simulink model "UAV_Dynamics_Autopilot_Communication_ver2023b"  (R2023b)
settings: Solver=ode4  StartTime=0.0  StopTime=inf  FixedStep=1/1000  RelTol=1e-3
values from neighbouring files (symbols this model uses):
  dragCoeffMov = 0.01    [InitHexacopterPlantVars.m]
  m_to_mm = 1000    [InitHexacopterPlantVars.m]
  ms_to_cms = 100    [InitHexacopterPlantVars.m]
  ref_height = 23    [InitHexacopterPlantVars.m]
  ref_lat = 36.364905    [InitHexacopterPlantVars.m]
  ref_lon = 127.344377    [InitHexacopterPlantVars.m]
  rotorDir = [1 -1 1 -1 -1 1]    [InitHexacopterPlantVars.m]
  rotorPositions = zeros(3,6)    [InitHexacopterPlantVars.m]
  rotorThrustMax = 4    [InitHexacopterPlantVars.m]
  rotorTimeConst = 0.050    (= 0.05)    [InitHexacopterPlantVars.m]
  rotorTorqueMax = 0.05    [InitHexacopterPlantVars.m]
  SampleTime = 1/100    (= 0.01)    [InitHexacopterPlantVars.m]
  Ts_sensor = 1/100    (= 0.01)    [InitHexacopterPlantVars.m]
  uT_to_gauss = 0.01    [InitHexacopterPlantVars.m]
  windVel = [0 0 0]'    [InitHexacopterPlantVars.m]
  x0 = [0 0 0 0 0 0 0 0 0 0 0 0]    [InitHexacopterPlantVars.m]
undefined symbols (not defined in the file or in its folder): contact, control, ddx, ddy, ddz, dx, dy, dz, earthRadius, fractalcoef, g, Mass, p, Payload, pitch, q, r, r2d, Receive, roll, Send, X, Y, yaw, Z
libraries: uavmavlinklib x7, aerolibfltsims x3, px4MAVLinkBridgelib x2, aerolibanimutils x2, aerolibatmos2 x1, sensorgpslib x1, robotcorelib x1, mspsensorlib x1, shared6dof x1, simulink x1
settings Model: Creator=The MathWorks, Inc.  LastModifiedBy=CNU_UASG
settings SolverCC: MaxZcPerStep=1
settings ModelReferenceCC: EnableRefExpFcnMdlSchedulingChecks=on
settings RTWCC: DLArmComputeVersion=19.05

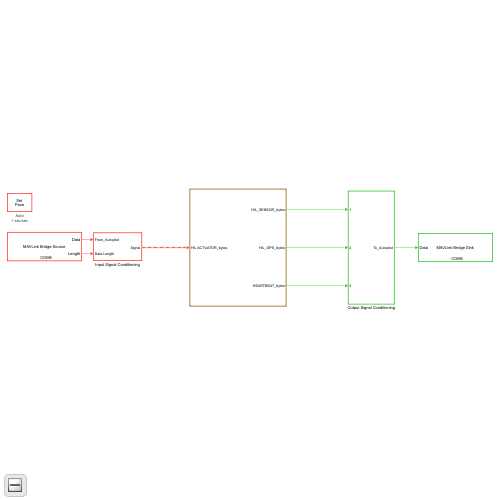
[thumbnail: Simulink's stored preview of the top-level diagram]
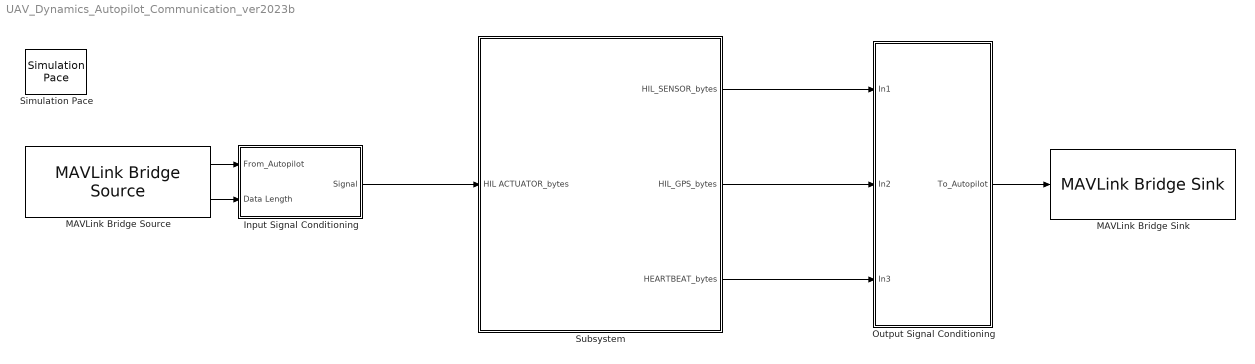
== system UAV_Dynamics_Autopilot_Communication_ver2023b ==
  Input Signal Conditioning : Subsystem
  MAVLink Bridge Sink : px4MAVLinkBridgelib/MAVLink Bridge Sink  PixhawkSerialPorttemp=Specify manually  PixhawkSerialPortManually=COM6  FieldTable={ 'UDP', '127.0.0.1', '14550' }
  MAVLink Bridge Source : px4MAVLinkBridgelib/MAVLink Bridge Source  PixhawkSerialPorttemp=Specify manually  PixhawkSerialPortManually=COM6  dataLength=MAVLink_Input_Read_Size  FieldTable={ 'UDP', '127.0.0.1', '14550' }  SampleTime=-1
  Output Signal Conditioning : Subsystem
  Simulation Pace : aerolibanimutils/Simulation Pace  SimulationPace=1  SleepMode=Auto  OutputPaceError=off  SampleTime=-1
  Subsystem : Subsystem
  wires:
  Subsystem/2(HIL_GPS_bytes) -> Output Signal Conditioning/2(In2)
  Subsystem/1(HIL_SENSOR_bytes) -> Output Signal Conditioning/1(In1)
  Subsystem/3(HEARTBEAT_bytes) -> Output Signal Conditioning/3(In3)
  Input Signal Conditioning/1(Signal) -> Subsystem/1(HIL ACTUATOR_bytes)
  MAVLink Bridge Source/1 -> Input Signal Conditioning/1(From_Autopilot)
  MAVLink Bridge Source/2 -> Input Signal Conditioning/2(Data Length)
  Output Signal Conditioning/1(To_Autopilot) -> MAVLink Bridge Sink/1

== system UAV_Dynamics_Autopilot_Communication_ver2023b/Input Signal Conditioning ==
  From_Autopilot : Inport
  Data Length : Inport  Port=2
  Constant : Constant
  Constant1 : Constant  Value=0  OutDataTypeStr=uint8  SampleTime=-1
  Data Type Conversion : DataTypeConversion  OutDataTypeStr=double  SaturateOnIntegerOverflow=off  RndMeth=Floor
  Mux1 : Mux  Inputs=2
  Reshape : Reshape
  Selector : Selector  InputPortWidth=MAVLink_Input_Read_Size  IndexOptions=Starting and ending indices (port)  Indices=[1 3]  OutputSizes=1
  Switch : Switch  Criteria=u2 > Threshold  SaturateOnIntegerOverflow=off  InputSameDT=off
  Signal : Outport
  wires:
  Reshape/1 -> Signal/1
  Mux1/1 -> Selector/2
  Data Length/1 -> Data Type Conversion/1
  Constant/1 -> Mux1/1
  Selector/1 -> Switch/1
  From_Autopilot/1 -> Selector/1
  Constant1/1 -> Switch/3
  Switch/1 -> Reshape/1
  Data Type Conversion/1 -> Switch/2, Mux1/2

== system UAV_Dynamics_Autopilot_Communication_ver2023b/Output Signal Conditioning ==
  In1 : Inport
  In2 : Inport  Port=2
  In3 : Inport  Port=3
  Mux : Mux  Inputs=3
  To_Autopilot : Outport
  wires:
  Mux/1 -> To_Autopilot/1
  In2/1 -> Mux/2
  In3/1 -> Mux/3
  In1/1 -> Mux/1

== system UAV_Dynamics_Autopilot_Communication_ver2023b/Subsystem ==
  HIL ACTUATOR_bytes : Inport  OutDataTypeStr=uint8  PortDimensions=MAVLink_Input_Read_Size  SampleTime=SampleTime  Interpolate=off
      settings: VarSizeSig=Yes
  HIL_ACTUATOR_CONTROLS : Subsystem
  HIL_GPS : Subsystem
  HIL_SENSOR : Subsystem
  Send Heartbeat : Subsystem
  Subsystem : Subsystem
  HIL_SENSOR_bytes : Outport  BusOutputAsStruct=on
  HIL_GPS_bytes : Outport  Port=2  BusOutputAsStruct=on
  HEARTBEAT_bytes : Outport  Port=3  BusOutputAsStruct=on
  wires:
  Subsystem/2(Gyro) -> HIL_SENSOR/2(Gyro)
  Subsystem/4(Pressure) -> HIL_SENSOR/4(Pressure)
  Subsystem/6(Velocity) -> HIL_GPS/2(Velocity)
  Subsystem/3(Mag) -> HIL_SENSOR/3(Mag)
  Subsystem/8(Course) -> HIL_GPS/4(Course)
  HIL_ACTUATOR_CONTROLS/1(Actuator) -> Subsystem/1(PWM Inputs)
  Subsystem/1(Acc) -> HIL_SENSOR/1(Acc)
  Subsystem/5(LLA) -> HIL_GPS/1(LLA)
  HIL_GPS/1(HIL_GPS_bytes) -> HIL_GPS_bytes/1
  HIL_SENSOR/1(HIL_SENSOR_bytes) -> HIL_SENSOR_bytes/1
  HIL ACTUATOR_bytes/1 -> HIL_ACTUATOR_CONTROLS/1(HIL ACTUATOR_bytes)
  Subsystem/7(GndSpeed) -> HIL_GPS/3(GndSpeed)
  Send Heartbeat/1(HEARTBEAT_bytes) -> HEARTBEAT_bytes/1

== system UAV_Dynamics_Autopilot_Communication_ver2023b/Subsystem/HIL_ACTUATOR_CONTROLS ==
  HIL ACTUATOR_bytes : Inport
  Bus Selector : BusSelector  OutputSignals=Payload.controls
  Data Type Conversion : DataTypeConversion  OutDataTypeStr=double  SaturateOnIntegerOverflow=off  RndMeth=Floor
  MAVLink Deserializer : uavmavlinklib/MAVLink Deserializer  dialectSource=Select from standard MAVLink dialects  dialect=common.xml  dialectCustom=common.xml  version=2  messageType=HIL_ACTUATOR_CONTROLS  inputDataLength=off  SystemIDFilter=off  systemID=1  ComponentIDFilter=off  componentID=1  queueMsg=off  queueMsgSize=50  dropNum=off
  Saturation : Saturate  UpperLimit=1  LowerLimit=0
  Selector1 : Selector  InputPortWidth=16  IndexOptions=Index vector (dialog)  Indices=[1:6]  OutputSizes=1
  Terminator : Terminator
  Actuator : Outport
  wires:
  Saturation/1 -> Actuator/1
  Selector1/1 -> Saturation/1  "Controls"
  HIL ACTUATOR_bytes/1 -> MAVLink Deserializer/1
  Bus Selector/1 -> Data Type Conversion/1  "<controls>"
  MAVLink Deserializer/2 -> Bus Selector/1
  MAVLink Deserializer/1 -> Terminator/1
  Data Type Conversion/1 -> Selector1/1

== system UAV_Dynamics_Autopilot_Communication_ver2023b/Subsystem/HIL_GPS ==
  LLA : Inport
  Velocity : Inport  Port=2
  GndSpeed : Inport  Port=3
  Course : Inport  Port=4
  HIL_GPS Subsystem : Subsystem
  MAVLink Serializer3 : uavmavlinklib/MAVLink Serializer  dialectSource=Select from standard MAVLink dialects  dialect=common.xml  dialectCustom=common.xml  version=2  messageType=HIL_GPS
  Rate Transition : RateTransition  OutPortSampleTime=Ts_sensor
  Terminator2 : Terminator
  HIL_GPS_bytes : Outport
  wires:
  Rate Transition/1 -> MAVLink Serializer3/1
  Velocity/1 -> HIL_GPS Subsystem/2(Velocity)
  MAVLink Serializer3/1 -> HIL_GPS_bytes/1
  GndSpeed/1 -> HIL_GPS Subsystem/3(GndSpeed)
  LLA/1 -> HIL_GPS Subsystem/1(LLA)
  MAVLink Serializer3/2 -> Terminator2/1
  Course/1 -> HIL_GPS Subsystem/4(Course)
  HIL_GPS Subsystem/1(Out1) -> Rate Transition/1

== system UAV_Dynamics_Autopilot_Communication_ver2023b/Subsystem/HIL_SENSOR ==
  Acc : Inport
  Gyro : Inport  Port=2
  Mag : Inport  Port=3
  Pressure : Inport  Port=4
  HIL_SENSOR Creation subsystem : Subsystem
  MAVLink Serializer1 : uavmavlinklib/MAVLink Serializer  dialectSource=Select from standard MAVLink dialects  dialect=common.xml  dialectCustom=common.xml  version=2  messageType=HIL_SENSOR
  Rate Transition : RateTransition  OutPortSampleTime=Ts_sensor
  Terminator : Terminator
  HIL_SENSOR_bytes : Outport
  wires:
  Rate Transition/1 -> MAVLink Serializer1/1
  Gyro/1 -> HIL_SENSOR Creation subsystem/2(Gyro)
  HIL_SENSOR Creation subsystem/1(HIL Sensor) -> Rate Transition/1
  Mag/1 -> HIL_SENSOR Creation subsystem/3(Mag)
  MAVLink Serializer1/1 -> HIL_SENSOR_bytes/1
  MAVLink Serializer1/2 -> Terminator/1
  Acc/1 -> HIL_SENSOR Creation subsystem/1(Acc)
  Pressure/1 -> HIL_SENSOR Creation subsystem/4(Pressure)

== system UAV_Dynamics_Autopilot_Communication_ver2023b/Subsystem/Send Heartbeat ==
  Bus Assignment : BusAssignment  AssignedSignals=Payload.autopilot,Payload.type
  Constant : Constant  SampleTime=-1
  Constant1 : Constant  Value=12  SampleTime=-1
  Data Type Conversion : DataTypeConversion  OutDataTypeStr=uint8  SaturateOnIntegerOverflow=off  RndMeth=Floor
  Data Type Conversion1 : DataTypeConversion  OutDataTypeStr=uint8  SaturateOnIntegerOverflow=off  RndMeth=Floor
  MAVLink Blank Message : uavmavlinklib/MAVLink Blank Message  dialectSource=Select from standard MAVLink dialects  dialect=common.xml  dialectCustom=common.xml  version=2  messageType=HEARTBEAT  SystemID=2  ComponentID=51  SampleTime=Ts_sensor
  MAVLink Serializer : uavmavlinklib/MAVLink Serializer  dialectSource=Select from standard MAVLink dialects  dialect=common.xml  dialectCustom=common.xml  version=2  messageType=HEARTBEAT
  Terminator4 : Terminator
  HEARTBEAT_bytes : Outport
  wires:
  MAVLink Blank Message/1 -> Bus Assignment/1
  Constant1/1 -> Data Type Conversion1/1
  MAVLink Serializer/2 -> Terminator4/1
  Data Type Conversion/1 -> Bus Assignment/2
  Data Type Conversion1/1 -> Bus Assignment/3
  MAVLink Serializer/1 -> HEARTBEAT_bytes/1
  Constant/1 -> Data Type Conversion/1
  Bus Assignment/1 -> MAVLink Serializer/1

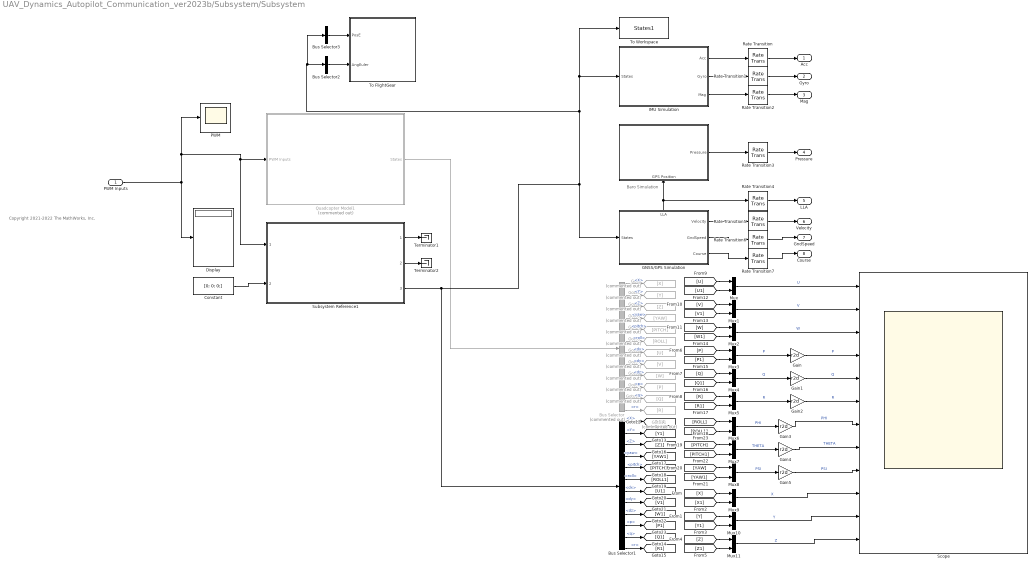
== system UAV_Dynamics_Autopilot_Communication_ver2023b/Subsystem/Subsystem ==
  note: Baro Simulation
  note: Copyright 2021-2022 The MathWorks, Inc.
  PWM Inputs : Inport
  " " : Subsystem
      settings: PortSchema="{\"entries\":[{\"content\":{\"sides\":[{\"content\":{\"connectorIds\":[]},\"type\":\"ConnectorPlacement.EquallySpacedRectSide\",\"uuid\":\"7ecc8b21-8f8f-4144-826a-6b68e30dbf7d\"},{\"content\":{\"connectorIds\":[\"Out1\"],\"side\":\"RIGHT\"},\"type\":\"ConnectorPlacement.EquallySpacedRectSide\",\"uuid\":\"81a1dd55-8330-4386-9921-36c0eb60d526\"},{\"content\":{\"connectorIds\":[],\"side\":\"TOP\"},\"type\":\"ConnectorPlacement.EquallySpacedRectSide\",\"uuid\":\"b99caff5-b40d-407d-b30e-35210c1aee1d\"},{\"content\":{\"connectorIds\":[\"In1\"],\"side\":\"BOTTOM\"},\"type\":\"ConnectorPlacement.EquallySpacedRectSide\",\"uuid\":\"18bfda3d-4fab-4e61-9ebc-e384e51de306\"}]},\"type\":\"ConnectorPlacement.EquallySpacedConnector\",\"uuid\":\"17ab4e96-b761-4c62-a0bb-ab626dac3eaa\"}],\"packageUris\":[\"http://schema.mathworks.com/mf0/Connector/R2020b\"],\"version\":\"1.0\"}"
  Bus Selector : BusSelector  Commented=on  OutputSignals=X,Y,Z,yaw,pitch,roll,dx,dy,dz,p,q,r
  Bus Selector1 : BusSelector  OutputSignals=X,Y,Z,yaw,pitch,roll,dx,dy,dz,p,q,r
  Bus Selector2 : BusSelector  OutputSignals=roll,pitch,yaw  OutputAsBus=on
  Bus Selector3 : BusSelector  OutputSignals=X,Y,Z  OutputAsBus=on
  Constant : Constant  Value=[0; 0; 0;]
  Display : Display
  GNSS/GPS Simulation : Subsystem
      settings: PortSchema="{\"entries\":[{\"content\":{\"sides\":[{\"content\":{\"connectorIds\":[\"In1\"]},\"type\":\"ConnectorPlacement.EquallySpacedRectSide\",\"uuid\":\"4934e8ff-5d4b-4e11-968d-c23bd62383a0\"},{\"content\":{\"connectorIds\":[\"Out1\",\"Out2\",\"Out3\"],\"side\":\"RIGHT\"},\"type\":\"ConnectorPlacement.EquallySpacedRectSide\",\"uuid\":\"9ec8bc0a-2d3c-4dca-835c-010ac29b6ebc\"},{\"content\":{\"connectorIds\":[\"Out4\"],\"side\":\"TOP\"},\"type\":\"ConnectorPlacement.EquallySpacedRectSide\",\"uuid\":\"04f09eb4-1bd9-450e-b951-47054bdd92ad\"}]},\"type\":\"ConnectorPlacement.EquallySpacedConnector\",\"uuid\":\"9a5920cf-a58d-4c98-839b-fbac94edbe7e\"}],\"packageUris\":[\"http://schema.mathworks.com/mf0/Connector/R2020b\"],\"version\":\"1.0\"}"
  Gain{,1..5} (6 alike) : Gain  Gain=r2d
  Goto : Goto  Commented=on  GotoTag=X
  Goto1 : Goto  Commented=on  GotoTag=Y
  Goto10 : Goto  Commented=on  GotoTag=Q
  Goto11 : Goto  Commented=on  GotoTag=R
  Goto2 : Goto  Commented=on  GotoTag=Z
  Goto3 : Goto  Commented=on  GotoTag=YAW
  Goto4 : Goto  Commented=on  GotoTag=PITCH
  Goto5 : Goto  Commented=on  GotoTag=ROLL
  Goto6 : Goto  Commented=on  GotoTag=U
  Goto7 : Goto  Commented=on  GotoTag=V
  Goto8 : Goto  Commented=on  GotoTag=W
  Goto9 : Goto  Commented=on  GotoTag=P
  IMU Simulation : Subsystem
  Mux{,1..11} (12 alike) : Mux  Inputs=2
  PWM : Scope
  Quadcopter Model1 : Subsystem  Commented=on
  Rate Transition{,1..7} (8 alike) : RateTransition  OutPortSampleTime=Ts_sensor
  Scope : Scope  NumInputPorts=12
  Subsystem Reference1 : Subsystem  ReferencedSubsystem=F550_Dynamics_sub_ver2023b
  Terminator1 : Terminator
  Terminator2 : Terminator
  To FlightGear : Subsystem
      mask Display: image('79904309.png');
  To Workspace : ToWorkspace  VariableName=States1  SaveFormat=Structure With Time  SampleTime=-1
  Acc : Outport
  Gyro : Outport  Port=2
  Mag : Outport  Port=3
  Pressure : Outport  Port=4
  LLA : Outport  Port=5
  Velocity : Outport  Port=6
  GndSpeed : Outport  Port=7
  Course : Outport  Port=8
  wires:
  Subsystem Reference1/1 -> Terminator1/1
  Bus Selector/8 -> Goto7/1  "<dy>"
  [PITCH1] -> Mux7/2
  Mux2/1 -> Scope/3  "W"
  Bus Selector1/1 -> [X1]  "<X>"
  GNSS/GPS Simulation/2(GndSpeed) -> Rate Transition6/1
  [YAW1] -> Mux8/2
  [X] -> Mux9/1
  GNSS/GPS Simulation/1(Velocity) -> Rate Transition5/1
  PWM Inputs/1 -> Display/1, PWM/1, Quadcopter Model1/1(PWM Inputs), Subsystem Reference1/1
  [PITCH] -> Mux7/1
  [YAW] -> Mux8/1
  [X1] -> Mux9/2
  Bus Selector/12 -> Goto11/1  "<r>"
  Bus Selector1/2 -> [Y1]  "<Y>"
  GNSS/GPS Simulation/3(Course) -> Rate Transition7/1
  Constant/1 -> Subsystem Reference1/2
  Bus Selector1/5 -> [PITCH1]  "<pitch>"
  Bus Selector/3 -> Goto2/1  "<Z>"
  Bus Selector/6 -> Goto5/1  "<roll>"
  Bus Selector1/4 -> [YAW1]  "<yaw>"
  Mux8/1 -> Gain5/1  "PSI"
  Bus Selector1/12 -> [R1]  "<r>"
  IMU Simulation/2(Gyro) -> Rate Transition1/1
  [P] -> Mux3/1
  [U1] -> Mux/2
  [Q1] -> Mux4/2
  [Y1] -> Mux10/2
  [Z] -> Mux11/1
  Bus Selector/11 -> Goto10/1  "<q>"
  Bus Selector/7 -> Goto6/1  "<dx>"
  Bus Selector/5 -> Goto4/1  "<pitch>"
  Bus Selector/1 -> Goto/1  "<X>"
  Bus Selector/4 -> Goto3/1  "<yaw>"
  Bus Selector1/10 -> [P1]  "<p>"
  [Z1] -> Mux11/2
  Bus Selector/10 -> Goto9/1  "<p>"
  [V1] -> Mux1/2
  Mux7/1 -> Gain4/1  "THETA"
  [R] -> Mux5/1
  " "/1(Pressure) -> Rate Transition3/1
  [W1] -> Mux2/2
  [P1] -> Mux3/2
  GNSS/GPS Simulation/4(LLA) -> " "/1(GPS Position), Rate Transition4/1
  [Q] -> Mux4/1
  Bus Selector1/8 -> [V1]  "<dy>"
  [Y] -> Mux10/1
  Bus Selector3/1 -> To FlightGear/1(PosE)
  Subsystem Reference1/2 -> Terminator2/1
  [V] -> Mux1/1
  [W] -> Mux2/1
  [ROLL] -> Mux6/1
  Mux/1 -> Scope/1  "U"
  Mux10/1 -> Scope/11  "Y"
  Bus Selector1/9 -> [W1]  "<dz>"
  [R1] -> Mux5/2
  Mux1/1 -> Scope/2  "V"
  Mux4/1 -> Gain1/1  "Q"
  Mux6/1 -> Gain3/1  "PHI"
  Mux3/1 -> Gain/1  "P"
  Mux9/1 -> Scope/10  "X"
  Bus Selector/2 -> Goto1/1  "<Y>"
  Bus Selector1/11 -> [Q1]  "<q>"
  Bus Selector1/6 -> [ROLL1]  "<roll>"
  [ROLL1] -> Mux6/2
  Mux11/1 -> Scope/12  "Z"
  IMU Simulation/1(Acc) -> Rate Transition/1
  IMU Simulation/3(Mag) -> Rate Transition2/1
  Bus Selector2/1 -> To FlightGear/2(AngEuler)
  [U] -> Mux/1
  Bus Selector1/3 -> [Z1]  "<Z>"
  Bus Selector/9 -> Goto8/1  "<dz>"
  Bus Selector1/7 -> [U1]  "<dx>"
  Quadcopter Model1/1(States) -> Bus Selector/1
  Mux5/1 -> Gain2/1  "R"
  Gain/1 -> Scope/4  "P"
  Gain1/1 -> Scope/5  "Q"
  Gain2/1 -> Scope/6  "R"
  Gain3/1 -> Scope/7  "PHI"
  Gain4/1 -> Scope/8  "THETA"
  Gain5/1 -> Scope/9  "PSI"
  Subsystem Reference1/3 -> GNSS/GPS Simulation/1(States), IMU Simulation/1(States), To Workspace/1, Bus Selector2/1, Bus Selector3/1, Bus Selector1/1
  Rate Transition/1 -> Acc/1
  Rate Transition1/1 -> Gyro/1
  Rate Transition2/1 -> Mag/1
  Rate Transition3/1 -> Pressure/1
  Rate Transition4/1 -> LLA/1
  Rate Transition5/1 -> Velocity/1
  Rate Transition7/1 -> Course/1
  Rate Transition6/1 -> GndSpeed/1

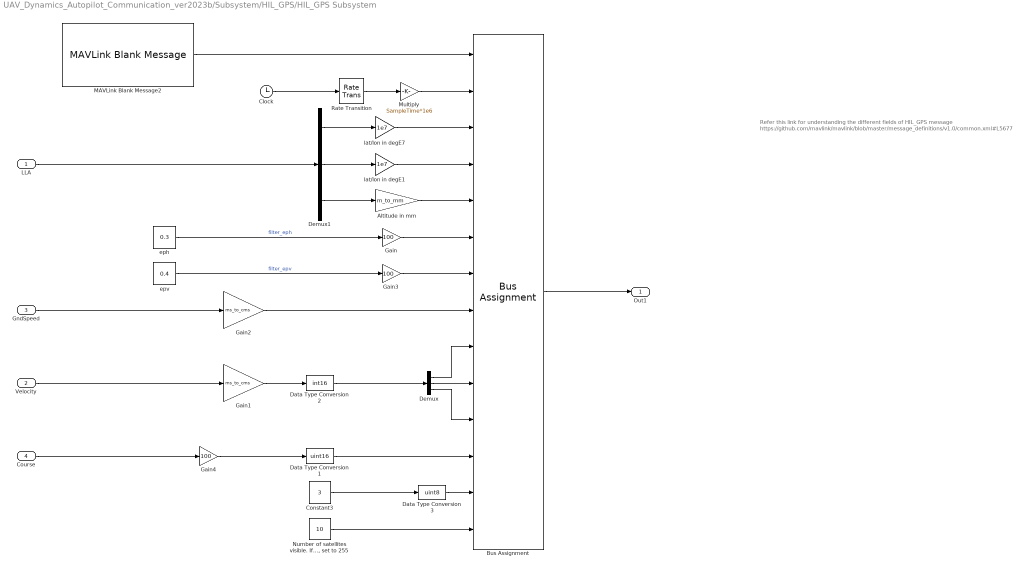
== system UAV_Dynamics_Autopilot_Communication_ver2023b/Subsystem/HIL_GPS/HIL_GPS Subsystem ==
  note: Refer this link for understanding the different fields of HIL_GPS message https://github.com/mavlink/mavlink/blob/master/message_definitions/v1.0/common.xml#L5677
  LLA : Inport
  Velocity : Inport  Port=2
  GndSpeed : Inport  Port=3
  Course : Inport  Port=4
  Altitude in mm : Gain  Gain=m_to_mm  OutDataTypeStr=Inherit: Inherit via back propagation
  Bus Assignment : BusAssignment  AssignedSignals=Payload.time_usec,Payload.lat,Payload.lon,Payload.alt,Payload.eph,Payload.epv,Payload.vel,Payload.vn,Payload.ve,Payload.vd,Payload.cog,Payload.fix_type,Payload.satellites_visible
  Clock : Clock
  Constant3 : Constant  Value=3  OutDataTypeStr=Inherit: Inherit via back propagation  SampleTime=Ts_sensor
  Data Type Conversion1 : DataTypeConversion  OutDataTypeStr=uint16  SaturateOnIntegerOverflow=off  RndMeth=Floor
  Data Type Conversion2 : DataTypeConversion  OutDataTypeStr=int16  SaturateOnIntegerOverflow=off  RndMeth=Floor
  Data Type Conversion3 : DataTypeConversion  OutDataTypeStr=uint8  SaturateOnIntegerOverflow=off  RndMeth=Floor
  Demux : Demux  Outputs=3
  Demux1 : Demux  Outputs=3
  Gain : Gain  Gain=100  OutDataTypeStr=Inherit: Inherit via back propagation
  Gain1 : Gain  Gain=ms_to_cms
  Gain2 : Gain  Gain=ms_to_cms  OutDataTypeStr=uint16
  Gain3 : Gain  Gain=100  OutDataTypeStr=Inherit: Inherit via back propagation
  Gain4 : Gain  Gain=100
  MAVLink Blank Message2 : uavmavlinklib/MAVLink Blank Message  dialectSource=Select from standard MAVLink dialects  dialect=common.xml  dialectCustom=common.xml  version=2  messageType=HIL_GPS  SystemID=2  ComponentID=51  SampleTime=Ts_sensor
  Multiply : Gain  Gain=SampleTime*1e6  OutDataTypeStr=Inherit: Inherit via back propagation
  "Number of satellites visible. If unknown, set to 255" : Constant  Value=10  OutDataTypeStr=Inherit: Inherit via back propagation  SampleTime=Ts_sensor
  Rate Transition : RateTransition  OutPortSampleTime=Ts_sensor
  eph : Constant  Value=0.3  SampleTime=Ts_sensor
  epv : Constant  Value=0.4  SampleTime=Ts_sensor
  lat/lon in degE1 : Gain  Gain=1e7  OutDataTypeStr=Inherit: Inherit via back propagation
  lat/lon in degE7 : Gain  Gain=1e7  OutDataTypeStr=Inherit: Inherit via back propagation
  Out1 : Outport
  wires:
  Multiply/1 -> Bus Assignment/2
  Rate Transition/1 -> Multiply/1
  Clock/1 -> Rate Transition/1
  Constant3/1 -> Data Type Conversion3/1
  Gain4/1 -> Data Type Conversion1/1
  Data Type Conversion3/1 -> Bus Assignment/13
  epv/1 -> Gain3/1  "filter_epv"
  eph/1 -> Gain/1  "filter_eph"
  Data Type Conversion1/1 -> Bus Assignment/12
  Course/1 -> Gain4/1
  Velocity/1 -> Gain1/1
  GndSpeed/1 -> Gain2/1
  LLA/1 -> Demux1/1
  Gain3/1 -> Bus Assignment/7
  Gain/1 -> Bus Assignment/6
  "Number of satellites visible. If unknown, set to 255"/1 -> Bus Assignment/14
  Bus Assignment/1 -> Out1/1
  Demux/2 -> Bus Assignment/10
  Data Type Conversion2/1 -> Demux/1
  Altitude in mm/1 -> Bus Assignment/5
  lat/lon in degE1/1 -> Bus Assignment/4
  Demux/1 -> Bus Assignment/9
  Demux1/2 -> lat/lon in degE1/1
  Demux1/3 -> Altitude in mm/1
  Gain1/1 -> Data Type Conversion2/1
  MAVLink Blank Message2/1 -> Bus Assignment/1
  Demux/3 -> Bus Assignment/11
  Demux1/1 -> lat/lon in degE7/1
  lat/lon in degE7/1 -> Bus Assignment/3
  Gain2/1 -> Bus Assignment/8

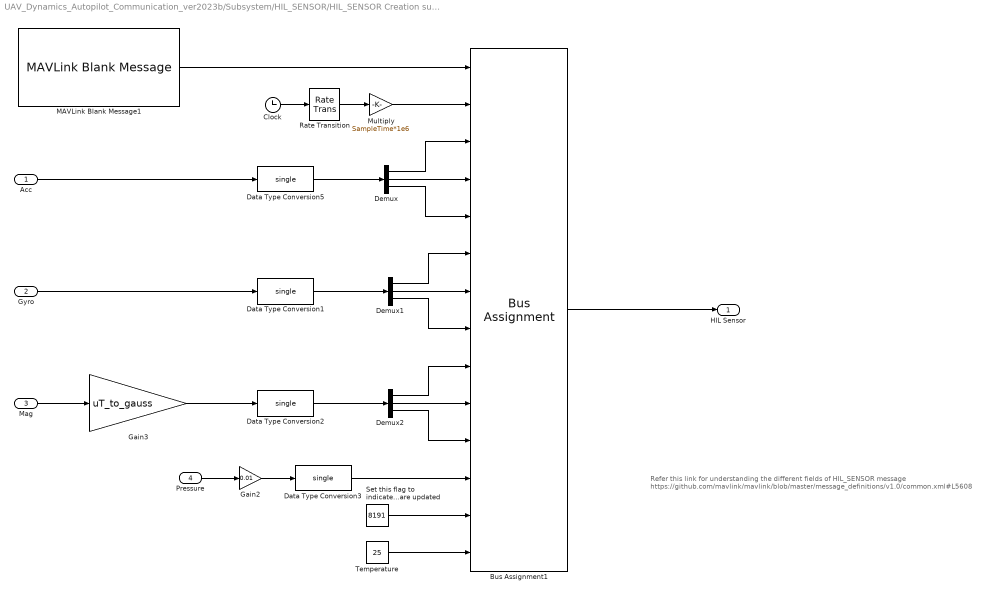
== system UAV_Dynamics_Autopilot_Communication_ver2023b/Subsystem/HIL_SENSOR/HIL_SENSOR Creation subsystem ==
  note: Refer this link for understanding the different fields of HIL_SENSOR message https://github.com/mavlink/mavlink/blob/master/message_definitions/v1.0/common.xml#L5608
  Acc : Inport
  Gyro : Inport  Port=2
  Mag : Inport  Port=3
  Pressure : Inport  Port=4
  Bus Assignment1 : BusAssignment  AssignedSignals=Payload.time_usec,Payload.xacc,Payload.yacc,Payload.zacc,Payload.xgyro,Payload.ygyro,Payload.zgyro,Payload.xmag,Payload.ymag,Payload.zmag,Payload.abs_pressure,Payload.fields_updated,Payload.temperature
  Clock : Clock
  Data Type Conversion{1..3,5} (4 alike) : DataTypeConversion  OutDataTypeStr=single  SaturateOnIntegerOverflow=off  RndMeth=Floor
  Demux : Demux  Outputs=3
  Demux1 : Demux  Outputs=3
  Demux2 : Demux  Outputs=3
  Gain2 : Gain  Gain=0.01  OutDataTypeStr=single
  Gain3 : Gain  Gain=uT_to_gauss
  MAVLink Blank Message1 : uavmavlinklib/MAVLink Blank Message  dialectSource=Select from standard MAVLink dialects  dialect=common.xml  dialectCustom=common.xml  version=2  messageType=HIL_SENSOR  SystemID=2  ComponentID=51  SampleTime=Ts_sensor
  Multiply : Gain  Gain=SampleTime*1e6  OutDataTypeStr=Inherit: Inherit via back propagation
  Rate Transition : RateTransition  OutPortSampleTime=Ts_sensor
  Set this flag to indicate all flags are updated : Constant  Value=8191  OutDataTypeStr=Inherit: Inherit via back propagation  SampleTime=Ts_sensor
  Temperature : Constant  Value=25  OutDataTypeStr=Inherit: Inherit via back propagation  SampleTime=Ts_sensor
  HIL Sensor : Outport
  wires:
  Temperature/1 -> Bus Assignment1/14
  Gain2/1 -> Data Type Conversion3/1
  Multiply/1 -> Bus Assignment1/2
  Rate Transition/1 -> Multiply/1
  Clock/1 -> Rate Transition/1
  Pressure/1 -> Gain2/1
  Set this flag to indicate all flags are updated/1 -> Bus Assignment1/13
  Gain3/1 -> Data Type Conversion2/1
  Data Type Conversion3/1 -> Bus Assignment1/12
  Acc/1 -> Data Type Conversion5/1
  Demux1/2 -> Bus Assignment1/7
  Demux/2 -> Bus Assignment1/4
  Demux2/1 -> Bus Assignment1/9
  MAVLink Blank Message1/1 -> Bus Assignment1/1
  Demux/1 -> Bus Assignment1/3
  Data Type Conversion5/1 -> Demux/1
  Demux2/3 -> Bus Assignment1/11
  Demux2/2 -> Bus Assignment1/10
  Demux/3 -> Bus Assignment1/5
  Bus Assignment1/1 -> HIL Sensor/1
  Gyro/1 -> Data Type Conversion1/1
  Data Type Conversion1/1 -> Demux1/1
  Demux1/3 -> Bus Assignment1/8
  Mag/1 -> Gain3/1
  Demux1/1 -> Bus Assignment1/6
  Data Type Conversion2/1 -> Demux2/1

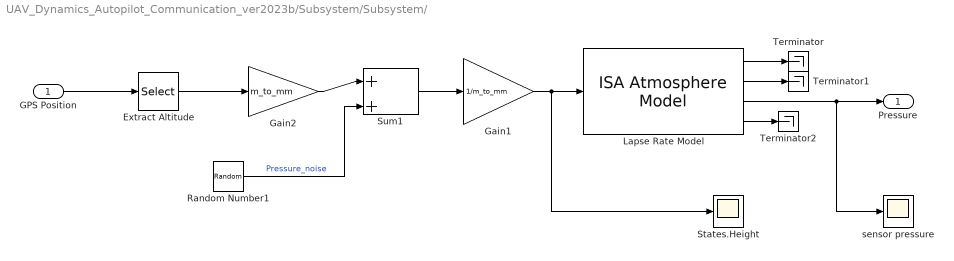
== system UAV_Dynamics_Autopilot_Communication_ver2023b/Subsystem/Subsystem/  ==
  GPS Position : Inport
  Extract Altitude : Selector  InputPortWidth=3  IndexOptions=Index vector (dialog)  Indices=[3]  OutputSizes=1
  Gain1 : Gain  Gain=1/m_to_mm
  Gain2 : Gain  Gain=m_to_mm
  Lapse Rate Model : aerolibatmos2/ISA Atmosphere Model  useExtended=off  action=Warning  custom=on  viscosityOut=off  g=9.80665  gamma=1.4  R=287.0531  L=0.0065  h_trop=11000  h_strat=20000  rho0=1.225  P0=101325  T0=288.15  h0=0
  Random Number1 : RandomNumber  Variance=10000  Seed=10
  States.Height : Scope
  Sum1 : Sum  Inputs=|++
  Terminator : Terminator
  Terminator1 : Terminator
  Terminator2 : Terminator
  sensor pressure : Scope
  Pressure : Outport
  wires:
  Random Number1/1 -> Sum1/2  "Pressure_noise"
  GPS Position/1 -> Extract Altitude/1
  Gain1/1 -> States.Height/1, Lapse Rate Model/1
  Extract Altitude/1 -> Gain2/1
  Gain2/1 -> Sum1/1
  Sum1/1 -> Gain1/1
  Lapse Rate Model/3 -> sensor pressure/1, Pressure/1
  Lapse Rate Model/1 -> Terminator/1
  Lapse Rate Model/4 -> Terminator2/1
  Lapse Rate Model/2 -> Terminator1/1

== system UAV_Dynamics_Autopilot_Communication_ver2023b/Subsystem/Subsystem/GNSS//GPS Simulation ==
  States : Inport
  Bus Selector : BusSelector  OutputSignals=dx,dy,dz  OutputAsBus=on
  Bus Selector1 : BusSelector  OutputSignals=X,Y,Z  OutputAsBus=on
  GPS : sensorgpslib/GPS  DispRefFrame=NED  PositionInputFormat=Local  ReferenceLocation=[ref_lat ref_lon ref_height]  HorizontalPositionAccuracy=0.01  VerticalPositionAccuracy=0.01  VelocityAccuracy=0.01  DecayFactor=0.99  SeedDouble=67  SimulateUsing=Code generation
  Reshape1 : Reshape  OutputDimensionality=Row vector (2-D)
  Reshape3 : Reshape  OutputDimensionality=Row vector (2-D)
  Velocity : Outport
  GndSpeed : Outport  Port=2
  Course : Outport  Port=3
  LLA : Outport  Port=4
  wires:
  GPS/4 -> Course/1
  GPS/3 -> GndSpeed/1
  States/1 -> Bus Selector1/1, Bus Selector/1
  GPS/2 -> Velocity/1
  Reshape1/1 -> GPS/2
  Bus Selector/1 -> Reshape1/1
  Bus Selector1/1 -> Reshape3/1
  GPS/1 -> LLA/1  "lla"
  Reshape3/1 -> GPS/1

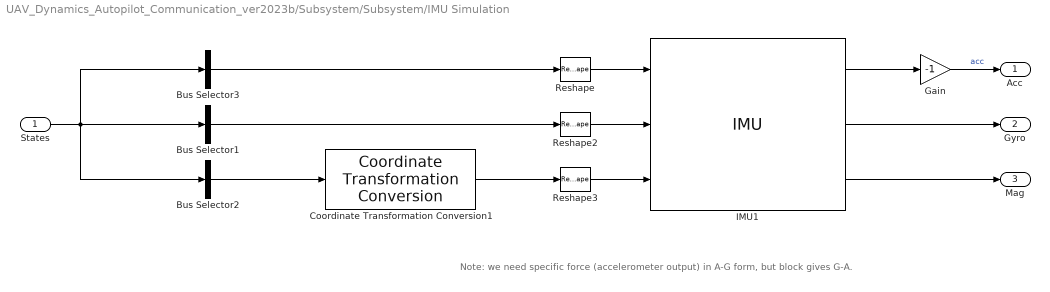
== system UAV_Dynamics_Autopilot_Communication_ver2023b/Subsystem/Subsystem/IMU Simulation ==
  note: Note:
      | we need specific force (accelerometer output) in A-G form, but block gives G-A.
  States : Inport
  Bus Selector1 : BusSelector  OutputSignals=p,q,r  OutputAsBus=on
  Bus Selector2 : BusSelector  OutputSignals=yaw,pitch,roll  OutputAsBus=on
  Bus Selector3 : BusSelector  OutputSignals=ddx,ddy,ddz  OutputAsBus=on
  Coordinate Transformation Conversion1 : robotcorelib/Coordinate Transformation Conversion  InputRepresentation=Euler Angles  InputEulerSequence=ZYX  ShowTrVecInputPort=on  OutputRepresentation=Quaternion  OutputEulerSequence=ZYX  ShowTrVecOutputPort=on  SimulateUsing=Code generation
  Gain : Gain  Gain=-1
  IMU1 : mspsensorlib/IMU  DispRefFrame=NED  TemperaturePort=off  Temperature=25  MagneticFieldPort=off  MagneticFieldNED=[21.5 1.16 43.1]  MagneticFieldENU=[ -2.4169, 27.5550, 16.0849 ]  SeedDouble=87254  SimulateUsing=Code generation  AccelParamsMeasurementRange=Inf  AccelParamsResolution=0  AccelParamsConstantBias=[ 0, 0, 0 ]  AccelParamsAxesMisalignment=[ 0, 0, 0 ]  AccelParamsNoiseDensity=0  AccelParamsBiasInstability=[ 0, 0, 0 ]  AccelParamsBiasInstabilityNumerator=fractalcoef().Numerator  AccelParamsBiasInstabilityDenominator=fractalcoef().Denominator  AccelParamsRandomWalk=[ 0, 0, 0 ]  AccelParamsNoiseType=double-sided  AccelParamsTemperatureBias=[ 0, 0, 0 ]  AccelParamsTemperatureScaleFactor=[ 0, 0, 0 ]  GyroParamsMeasurementRange=Inf  GyroParamsResolution=0  GyroParamsConstantBias=[ 0, 0, 0 ]  GyroParamsAxesMisalignment=[ 0, 0, 0 ]  GyroParamsAccelerationBias=0  GyroParamsNoiseDensity=0  GyroParamsBiasInstability=[ 0, 0, 0 ]  GyroParamsBiasInstabilityNumerator=fractalcoef().Numerator  GyroParamsBiasInstabilityDenominator=fractalcoef().Denominator  GyroParamsRandomWalk=[ 0, 0, 0 ]  GyroParamsNoiseType=double-sided  GyroParamsTemperatureBias=[ 0, 0, 0 ]  GyroParamsTemperatureScaleFactor=[ 0, 0, 0 ]  MagParamsMeasurementRange=Inf  MagParamsResolution=0  MagParamsConstantBias=[ 0, 0, 0 ]  MagParamsAxesMisalignment=[ 0, 0, 0 ]  MagParamsNoiseDensity=0  MagParamsBiasInstability=[ 0, 0, 0 ]  MagParamsBiasInstabilityNumerator=fractalcoef().Numerator  MagParamsBiasInstabilityDenominator=fractalcoef().Denominator  MagParamsRandomWalk=[ 0, 0, 0 ]  MagParamsNoiseType=double-sided  MagParamsTemperatureBias=[ 0, 0, 0 ]  MagParamsTemperatureScaleFactor=[ 0, 0, 0 ]
  Reshape : Reshape  OutputDimensionality=Row vector (2-D)
  Reshape2 : Reshape  OutputDimensionality=Row vector (2-D)
  Reshape3 : Reshape  OutputDimensionality=Row vector (2-D)
  Acc : Outport
  Gyro : Outport  Port=2
  Mag : Outport  Port=3
  wires:
  Gain/1 -> Acc/1  "acc"
  States/1 -> Bus Selector3/1, Bus Selector2/1, Bus Selector1/1
  Reshape2/1 -> IMU1/2
  Bus Selector2/1 -> Coordinate Transformation Conversion1/1
  Bus Selector1/1 -> Reshape2/1
  IMU1/1 -> Gain/1
  Bus Selector3/1 -> Reshape/1
  Reshape/1 -> IMU1/1
  IMU1/2 -> Gyro/1
  IMU1/3 -> Mag/1
  Reshape3/1 -> IMU1/3
  Coordinate Transformation Conversion1/1 -> Reshape3/1

== system UAV_Dynamics_Autopilot_Communication_ver2023b/Subsystem/Subsystem/Quadcopter Model1 ==
  note: Based on jmavsim quadcopter model
  note: Note:
      | DCM_be converts a vector written in earth frame to body frame
      | Abe is acceleration of body written in body frame, but measured relative to earth.
      | To get acceleration of body written in earth frame (NED fixed on takeoff location), we need to convert the frame.
      | IMU block's angular velocity and acceleration inputs are written in earth frame (NED)
  PWM Inputs : Inport
  "6DOF Rigid body dynamics " : shared6dof/6DOF (Euler Angles)  units=Metric (MKS)  mtype=Fixed  rep=Quaternion  xme_0=x0(10:12)  Vm_0=x0(1:3)  eul_0=x0(7:9)  pm_0=x0(4:6)  mass_0=Mass  mass_e=0.5  mass_f=2.0  inertia=Inertia  inertia_e=eye(3)  inertia_f=2*eye(3)  k_quat=1  vre_flag=on  abi_flag=on  aMode=aMode  xme_statename=''  Vm_statename=''  eul_statename=''  quat_statename=''  pm_statename=''  mass_statename=''
  Create States Bus : Subsystem
  Force and Moment Calculation : Subsystem
  Matrix Multiply : Product  Multiplication=Matrix(*)
  Matrix Multiply1 : Product  Multiplication=Matrix(*)
  Terminator1 : Terminator
  Terminator2 : Terminator
  Transpose : Math  Operator=transpose
  ypr : Selector  InputPortWidth=3  IndexOptions=Index vector (dialog)  Indices=[3 2 1]  OutputSizes=1
  States : Outport
  wires:
  Matrix Multiply1/1 -> Create States Bus/5(acc_lnav)
  "6DOF Rigid body dynamics "/4 -> Transpose/1, Force and Moment Calculation/1(DCMbe)
  Force and Moment Calculation/2(M_xyz) -> "6DOF Rigid body dynamics "/2
  "6DOF Rigid body dynamics "/8 -> Terminator2/1
  "6DOF Rigid body dynamics "/1 -> Create States Bus/1(Ve)
  "6DOF Rigid body dynamics "/7 -> Terminator1/1
  Create States Bus/1(States) -> States/1
  "6DOF Rigid body dynamics "/3 -> ypr/1, Force and Moment Calculation/5(rpy)
  "6DOF Rigid body dynamics "/2 -> Create States Bus/2(Xe), Force and Moment Calculation/3(Xe)
  ypr/1 -> Create States Bus/4(ypr)
  "6DOF Rigid body dynamics "/5 -> Force and Moment Calculation/2(Vb)
  Transpose/1 -> Matrix Multiply/1, Matrix Multiply1/1
  "6DOF Rigid body dynamics "/9 -> Matrix Multiply1/2
  Force and Moment Calculation/1(F_xyz) -> "6DOF Rigid body dynamics "/1
  "6DOF Rigid body dynamics "/6 -> Force and Moment Calculation/6(wb), Matrix Multiply/2
  Matrix Multiply/1 -> Create States Bus/3(pqr)
  PWM Inputs/1 -> Force and Moment Calculation/4(Inputs [0-1])

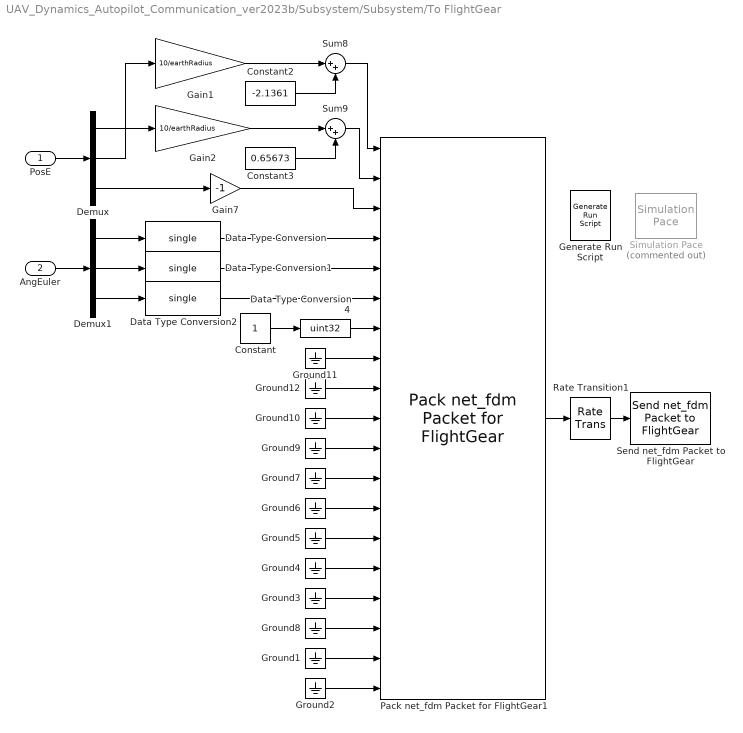
== system UAV_Dynamics_Autopilot_Communication_ver2023b/Subsystem/Subsystem/To FlightGear ==
  PosE : Inport
  AngEuler : Inport  Port=2
  Constant : Constant
  Constant2 : Constant  Value=-2.1361  VectorParams1D=off
  Constant3 : Constant  Value=0.65673  VectorParams1D=off
  Data Type Conversion : DataTypeConversion  OutDataTypeStr=single  RndMeth=Floor
  Data Type Conversion1 : DataTypeConversion  OutDataTypeStr=single  RndMeth=Floor
  Data Type Conversion2 : DataTypeConversion  OutDataTypeStr=single  RndMeth=Floor
  Data Type Conversion4 : DataTypeConversion  OutDataTypeStr=uint32  SaturateOnIntegerOverflow=off  RndMeth=Floor
  Demux : Demux  Outputs=3
  Demux1 : Demux  Outputs=3
  Gain1 : Gain  Gain=10/earthRadius
  Gain2 : Gain  Gain=10/earthRadius
  Gain7 : Gain  Gain=-1
  Generate Run Script : aerolibfltsims/Generate Run Script  Architecture=Default  dataFlow=Send-Receive  GeometryModelName=Rotor4  AirportId=KSF0  RunwayId=10L  InitialAltitude=0  InitialHeading=0  OffsetDistance=0  OffsetAzimuth=0  InstallScenery=off  DisableShaders=off  OriginAddress=127.0.0.1  DestinationPort=5502  OriginPort=5505  LocalAddress=127.0.0.1  OutputFileName=runfg.bat  FlightGearBaseDirectory=C:\Program Files\FlightGear 2016.1.2
  Ground{1..12} (12 alike) : Ground
  Pack net_fdm Packet for FlightGear1 : aerolibfltsims/Pack net_fdm Packet for FlightGear  FlightGearVersion=v2016.1  ShowPositionAttitudeInputs=on  ShowVelocityAccelerationInputs=off  ShowControlSurfacePositionInputs=off  ShowEngineFuelInputs=on  ShowLandingGearInputs=off  ShowEnvironmentInputs=off  SampleTime=-1  packetVersion=24
  Rate Transition1 : RateTransition
  Send net_fdm Packet to FlightGear : aerolibfltsims/Send net_fdm Packet to FlightGear  DestinationIpAddress=127.0.0.1  DestinationPort=5502  LocalIpPort=-1  varLen=off  SampleTime=0.01
  Simulation Pace : aerolibanimutils/Simulation Pace  Commented=on  SimulationPace=1  SleepMode=MATLAB Thread  OutputPaceError=off  SampleTime=-1
      settings: AttributesFormatString=%<SimulationPace> sec/sec
  Sum8 : Sum  Inputs=|++
  Sum9 : Sum  Inputs=|++
  wires:
  Ground12/1 -> Pack net_fdm Packet for FlightGear1/9
  Ground3/1 -> Pack net_fdm Packet for FlightGear1/16
  Ground4/1 -> Pack net_fdm Packet for FlightGear1/15
  Ground5/1 -> Pack net_fdm Packet for FlightGear1/14
  Ground6/1 -> Pack net_fdm Packet for FlightGear1/13
  Ground7/1 -> Pack net_fdm Packet for FlightGear1/12
  Ground9/1 -> Pack net_fdm Packet for FlightGear1/11
  Ground10/1 -> Pack net_fdm Packet for FlightGear1/10
  Ground11/1 -> Pack net_fdm Packet for FlightGear1/8
  Ground2/1 -> Pack net_fdm Packet for FlightGear1/19
  Ground1/1 -> Pack net_fdm Packet for FlightGear1/18
  Ground8/1 -> Pack net_fdm Packet for FlightGear1/17
  Gain7/1 -> Pack net_fdm Packet for FlightGear1/3
  Constant3/1 -> Sum9/2
  Constant2/1 -> Sum8/2
  Rate Transition1/1 -> Send net_fdm Packet to FlightGear/1
  Demux/2 -> Gain1/1
  Demux1/3 -> Data Type Conversion2/1
  Gain1/1 -> Sum8/1
  Gain2/1 -> Sum9/1
  Pack net_fdm Packet for FlightGear1/1 -> Rate Transition1/1
  Demux1/2 -> Data Type Conversion1/1
  Data Type Conversion4/1 -> Pack net_fdm Packet for FlightGear1/7
  Data Type Conversion2/1 -> Pack net_fdm Packet for FlightGear1/6
  Data Type Conversion1/1 -> Pack net_fdm Packet for FlightGear1/5
  Data Type Conversion/1 -> Pack net_fdm Packet for FlightGear1/4
  Sum8/1 -> Pack net_fdm Packet for FlightGear1/1
  Sum9/1 -> Pack net_fdm Packet for FlightGear1/2
  Demux/3 -> Gain7/1
  Constant/1 -> Data Type Conversion4/1
  Demux/1 -> Gain2/1
  Demux1/1 -> Data Type Conversion/1
  PosE/1 -> Demux/1
  AngEuler/1 -> Demux1/1

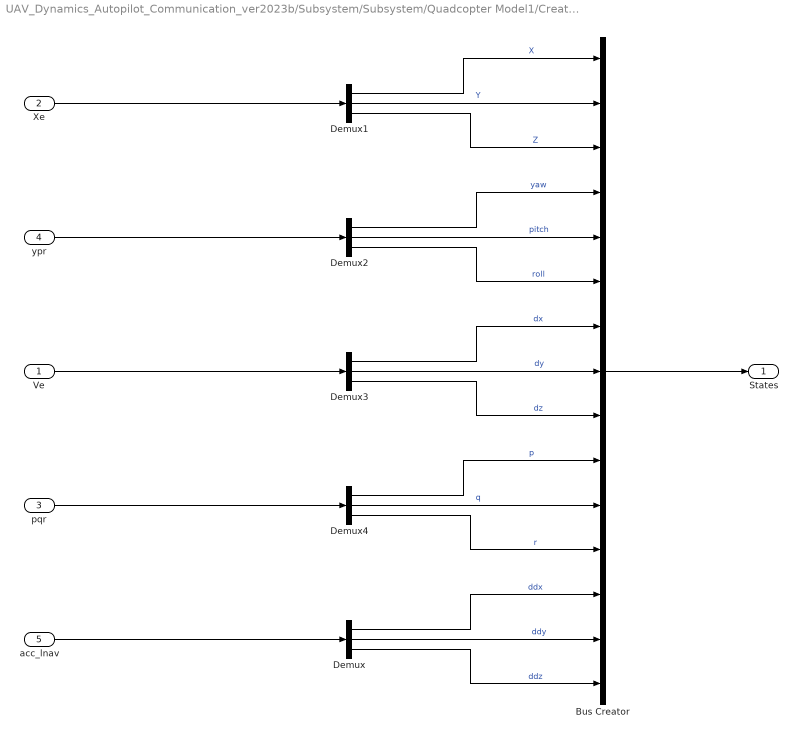
== system UAV_Dynamics_Autopilot_Communication_ver2023b/Subsystem/Subsystem/Quadcopter Model1/Create States Bus ==
  Ve : Inport
  Xe : Inport  Port=2
  pqr : Inport  Port=3
  ypr : Inport  Port=4
  acc_lnav : Inport  Port=5
  Bus Creator : BusCreator  Inputs=X,Y,Z,yaw,pitch,roll,dx,dy,dz,p,q,r,ddx,ddy,ddz
  Demux{,1..4} (5 alike) : Demux  Outputs=3
  States : Outport
  wires:
  Demux/1 -> Bus Creator/13  "ddx"
  Demux/2 -> Bus Creator/14  "ddy"
  Demux/3 -> Bus Creator/15  "ddz"
  acc_lnav/1 -> Demux/1
  Xe/1 -> Demux1/1
  Bus Creator/1 -> States/1
  Demux4/1 -> Bus Creator/10  "p"
  Demux4/3 -> Bus Creator/12  "r"
  Demux3/3 -> Bus Creator/9  "dz"
  Demux4/2 -> Bus Creator/11  "q"
  Demux3/1 -> Bus Creator/7  "dx"
  Demux1/3 -> Bus Creator/3  "Z"
  Demux2/1 -> Bus Creator/4  "yaw"
  Ve/1 -> Demux3/1
  pqr/1 -> Demux4/1
  Demux2/3 -> Bus Creator/6  "roll"
  Demux3/2 -> Bus Creator/8  "dy"
  Demux2/2 -> Bus Creator/5  "pitch"
  ypr/1 -> Demux2/1
  Demux1/2 -> Bus Creator/2  "Y"
  Demux1/1 -> Bus Creator/1  "X"

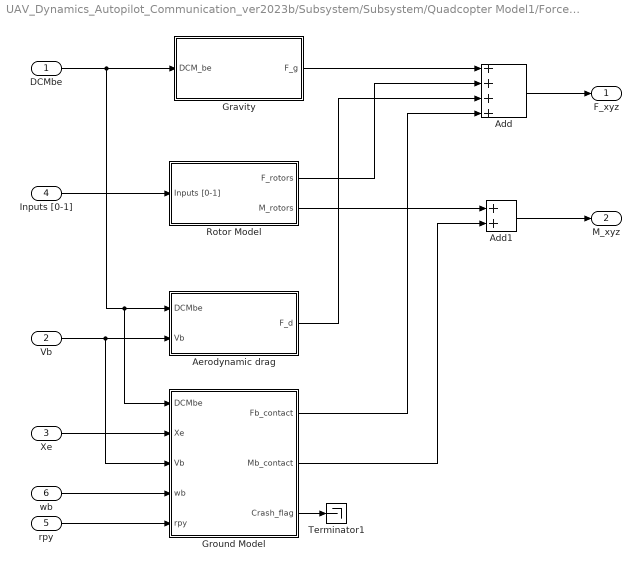
== system UAV_Dynamics_Autopilot_Communication_ver2023b/Subsystem/Subsystem/Quadcopter Model1/Force and Moment Calculation ==
  DCMbe : Inport
  Vb : Inport  Port=2
  Xe : Inport  Port=3
  Inputs [0-1] : Inport  Port=4
  rpy : Inport  Port=5
  wb : Inport  Port=6
  Add : Sum  Inputs=++++
  Add1 : Sum
  Aerodynamic drag : Subsystem
  Gravity : Subsystem
  Ground Model : Subsystem
  Rotor Model : Subsystem
  Terminator1 : Terminator
  F_xyz : Outport
  M_xyz : Outport  Port=2
  wires:
  Ground Model/3(Crash_flag) -> Terminator1/1
  Ground Model/1(Fb_contact) -> Add/4
  Add1/1 -> M_xyz/1
  Ground Model/2(Mb_contact) -> Add1/2
  Rotor Model/2(M_rotors) -> Add1/1
  rpy/1 -> Ground Model/5(rpy)
  wb/1 -> Ground Model/4(wb)
  Xe/1 -> Ground Model/2(Xe)
  Aerodynamic drag/1(F_d) -> Add/3
  Rotor Model/1(F_rotors) -> Add/2
  Vb/1 -> Aerodynamic drag/2(Vb), Ground Model/3(Vb)
  Add/1 -> F_xyz/1
  Gravity/1(F_g) -> Add/1
  DCMbe/1 -> Gravity/1(DCM_be), Aerodynamic drag/1(DCMbe), Ground Model/1(DCMbe)
  Inputs [0-1]/1 -> Rotor Model/1(Inputs [0-1])

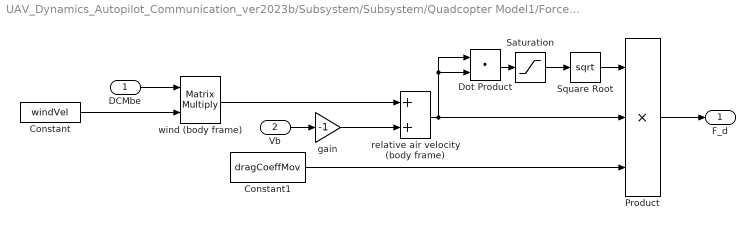
== system UAV_Dynamics_Autopilot_Communication_ver2023b/Subsystem/Subsystem/Quadcopter Model1/Force and Moment Calculation/Aerodynamic drag ==
  DCMbe : Inport
  Vb : Inport  Port=2
  Constant : Constant  Value=windVel
  Constant1 : Constant  Value=dragCoeffMov
  Dot Product : DotProduct  OutDataTypeStr=Inherit: Inherit via internal rule
  Product : Product  Inputs=3
  Saturation : Saturate  UpperLimit=inf  LowerLimit=0.0001
  Square Root : Sqrt
  gain : Gain  Gain=-1
  relative air velocity (body frame) : Sum
  wind (body frame) : Product  Multiplication=Matrix(*)
  F_d : Outport
  wires:
  Constant/1 -> wind (body frame)/2
  Constant1/1 -> Product/3
  gain/1 -> relative air velocity (body frame)/2
  wind (body frame)/1 -> relative air velocity (body frame)/1
  Square Root/1 -> Product/1
  Dot Product/1 -> Saturation/1
  Vb/1 -> gain/1
  Saturation/1 -> Square Root/1
  Product/1 -> F_d/1
  DCMbe/1 -> wind (body frame)/1
  relative air velocity (body frame)/1 -> Product/2, Dot Product/1, Dot Product/2

== system UAV_Dynamics_Autopilot_Communication_ver2023b/Subsystem/Subsystem/Quadcopter Model1/Force and Moment Calculation/Gravity ==
  DCM_be : Inport
  Constant : Constant  Value=[0 0 g]'
  Gain : Gain  Gain=Mass
  Matrix Multiply : Product  Multiplication=Matrix(*)
  F_g : Outport
  wires:
  Gain/1 -> F_g/1
  DCM_be/1 -> Matrix Multiply/1
  Constant/1 -> Matrix Multiply/2
  Matrix Multiply/1 -> Gain/1

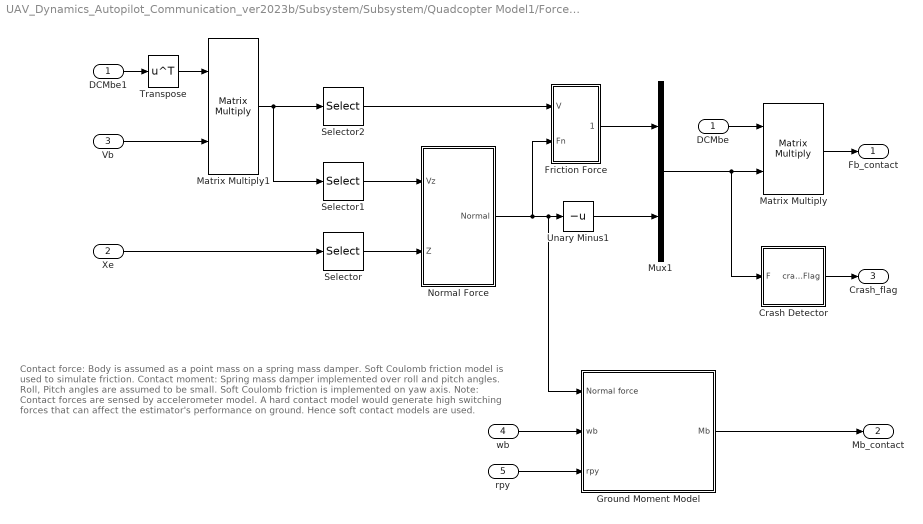
== system UAV_Dynamics_Autopilot_Communication_ver2023b/Subsystem/Subsystem/Quadcopter Model1/Force and Moment Calculation/Ground Model ==
  note: Contact force:
      | Body is assumed as a point mass on a spring mass damper. Soft Coulomb friction model is used to simulate friction.
      |
      | Contact moment:
      | Spring mass damper implemented over roll and pitch angles. Roll, Pitch angles are assumed to be small.
      | Soft Coulomb friction is implemented on yaw axis.
      |
      | Note:
      | Contact forces are sensed by accelerometer model. A hard contact model would generate high switching forces that can affect the estimator's performance on ground. Hence soft contact models are used.
  DCMbe : Inport
  Xe : Inport  Port=2
  Vb : Inport  Port=3
  wb : Inport  Port=4
  rpy : Inport  Port=5
  Crash Detector : Subsystem
  DCMbe1 : InportShadow
  Friction Force : Subsystem
  Ground Moment Model : Subsystem
  Matrix Multiply : Product  Multiplication=Matrix(*)
  Matrix Multiply1 : Product  Multiplication=Matrix(*)
  Mux1 : Mux  Inputs=2
  Normal Force : Subsystem
  Selector : Selector  InputPortWidth=3  IndexOptions=Index vector (dialog)  Indices=[3]  OutputSizes=1
  Selector1 : Selector  InputPortWidth=3  IndexOptions=Index vector (dialog)  Indices=[3]  OutputSizes=1
  Selector2 : Selector  InputPortWidth=3  IndexOptions=Index vector (dialog)  Indices=[1,2]  OutputSizes=1
  Transpose : Math  Operator=transpose
  Unary Minus1 : UnaryMinus
  Fb_contact : Outport
  Mb_contact : Outport  Port=2
  Crash_flag : Outport  Port=3
  wires:
  Ground Moment Model/1(Mb) -> Mb_contact/1
  rpy/1 -> Ground Moment Model/3(rpy)
  wb/1 -> Ground Moment Model/2(wb)
  Matrix Multiply1/1 -> Selector2/1, Selector1/1
  Vb/1 -> Matrix Multiply1/2
  Transpose/1 -> Matrix Multiply1/1
  DCMbe1/1 -> Transpose/1
  Friction Force/1(Friction) -> Mux1/1
  Selector2/1 -> Friction Force/1(V)
  Unary Minus1/1 -> Mux1/2
  Mux1/1 -> Matrix Multiply/2, Crash Detector/1(F)
  Normal Force/1(Normal) -> Friction Force/2(Fn), Unary Minus1/1, Ground Moment Model/1(Normal force)
  Matrix Multiply/1 -> Fb_contact/1
  DCMbe/1 -> Matrix Multiply/1
  Selector/1 -> Normal Force/2(Z)
  Selector1/1 -> Normal Force/1(Vz)
  Xe/1 -> Selector/1
  Crash Detector/1(crashFlag) -> Crash_flag/1

== system UAV_Dynamics_Autopilot_Communication_ver2023b/Subsystem/Subsystem/Quadcopter Model1/Force and Moment Calculation/Rotor Model ==
  Inputs [0-1] : Inport
  Constant : Constant  Value=rotorPositions
  Constant1 : Constant  Value=rotorDir
  MATLAB Function : MATLAB Function  TreatAsAtomicUnit=on
  Thrust model : Subsystem
  Torque model : Subsystem
  F_rotors : Outport
  M_rotors : Outport  Port=2
  wires:
  Thrust model/1(Out1) -> MATLAB Function/1(thrustEachRotor)
  Torque model/1(Out1) -> MATLAB Function/2(tauEachRotor)
  Constant1/1 -> MATLAB Function/4(rotorDir)
  Constant/1 -> MATLAB Function/3(rotorPositions)
  MATLAB Function/2(netM) -> M_rotors/1
  MATLAB Function/1(netF) -> F_rotors/1
  Inputs [0-1]/1 -> Thrust model/1(In1), Torque model/1(In1)

== system UAV_Dynamics_Autopilot_Communication_ver2023b/Subsystem/Subsystem/Quadcopter Model1/Force and Moment Calculation/Ground Model/Crash Detector ==
  F : Inport
  Compare To Constant : simulink/Logic and Bit Operations/Compare To Constant  relop=>  const=100  OutDataTypeStr=boolean
  Gain : Gain  Gain=1/Mass/g
  norm1 : Subsystem
  crashFlag : Outport
  wires:
  Gain/1 -> Compare To Constant/1  "g's"
  Compare To Constant/1 -> crashFlag/1
  norm1/1(Out1) -> Gain/1
  F/1 -> norm1/1(F)

== system UAV_Dynamics_Autopilot_Communication_ver2023b/Subsystem/Subsystem/Quadcopter Model1/Force and Moment Calculation/Ground Model/Friction Force ==
  V : Inport
  Fn : Inport  Port=2
  Product : Product
  Saturation : Saturate  UpperLimit=contact.translation.maxFriction  LowerLimit=-contact.translation.maxFriction
  Soft Coulomb Friction : Subsystem
  Unary Minus : UnaryMinus
  Friction : Outport
  wires:
  Saturation/1 -> Friction/1
  Unary Minus/1 -> Saturation/1
  V/1 -> Soft Coulomb Friction/1(In1)
  Product/1 -> Unary Minus/1
  Soft Coulomb Friction/1(Out1) -> Product/1
  Fn/1 -> Product/2

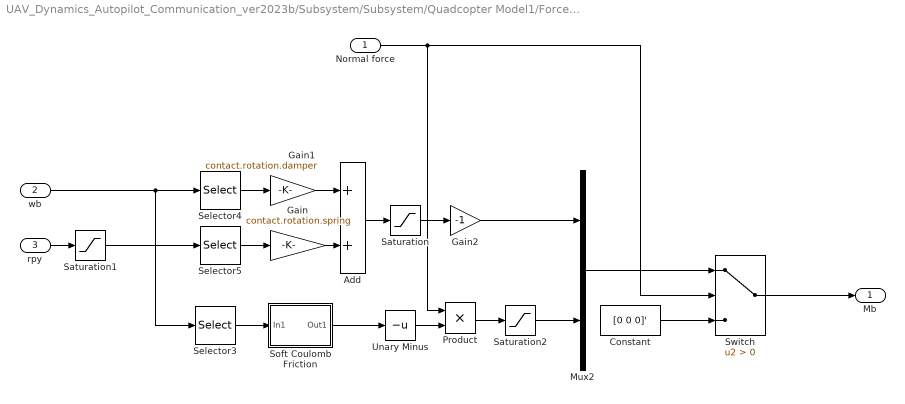
== system UAV_Dynamics_Autopilot_Communication_ver2023b/Subsystem/Subsystem/Quadcopter Model1/Force and Moment Calculation/Ground Model/Ground Moment Model ==
  Normal force : Inport
  wb : Inport  Port=2
  rpy : Inport  Port=3
  Add : Sum
  Constant : Constant  Value=[0 0 0]'
  Gain : Gain  Gain=contact.rotation.spring
  Gain1 : Gain  Gain=contact.rotation.damper
  Gain2 : Gain  Gain=-1
  Mux2 : Mux  Inputs=2
  Product : Product
  Saturation : Saturate  UpperLimit=control.rotation.maxMoment  LowerLimit=-control.rotation.maxMoment
  Saturation1 : Saturate  UpperLimit=20*pi/180  LowerLimit=-20*pi/180
  Saturation2 : Saturate  UpperLimit=control.rotation.maxMoment  LowerLimit=-control.rotation.maxMoment
  Selector3 : Selector  InputPortWidth=3  IndexOptions=Index vector (dialog)  Indices=[3]  OutputSizes=1
  Selector4 : Selector  InputPortWidth=3  IndexOptions=Index vector (dialog)  Indices=[1, 2]  OutputSizes=1
  Selector5 : Selector  InputPortWidth=3  IndexOptions=Index vector (dialog)  Indices=[1, 2]  OutputSizes=1
  Soft Coulomb Friction : Subsystem
  Switch : Switch  Criteria=u2 > Threshold  SaturateOnIntegerOverflow=off  InputSameDT=off
  Unary Minus : UnaryMinus
  Mb : Outport
  wires:
  Saturation2/1 -> Mux2/2
  Product/1 -> Saturation2/1
  Unary Minus/1 -> Product/2
  Soft Coulomb Friction/1(Out1) -> Unary Minus/1
  Selector3/1 -> Soft Coulomb Friction/1(In1)
  wb/1 -> Selector3/1, Selector4/1
  Saturation1/1 -> Selector5/1
  rpy/1 -> Saturation1/1
  Normal force/1 -> Switch/2, Product/1
  Mux2/1 -> Switch/1
  Switch/1 -> Mb/1
  Selector5/1 -> Gain/1
  Constant/1 -> Switch/3
  Gain1/1 -> Add/1
  Selector4/1 -> Gain1/1
  Saturation/1 -> Gain2/1
  Gain/1 -> Add/2
  Add/1 -> Saturation/1
  Gain2/1 -> Mux2/1

== system UAV_Dynamics_Autopilot_Communication_ver2023b/Subsystem/Subsystem/Quadcopter Model1/Force and Moment Calculation/Ground Model/Normal Force ==
  Vz : Inport
  Z : Inport  Port=2
  Add : Sum
  Constant : Constant  Value=0
  Damper Kp : Gain  Gain=-contact.translation.damper
  Saturation : Saturate  UpperLimit=contact.translation.maxNormal  LowerLimit=0
  Spring Kp : Gain  Gain=-contact.translation.spring
  Switch : Switch  Criteria=u2 > Threshold  SaturateOnIntegerOverflow=off  InputSameDT=off
  Unary Minus : UnaryMinus
  Unary Minus1 : UnaryMinus
  Normal : Outport
  wires:
  Unary Minus1/1 -> Damper Kp/1
  Unary Minus/1 -> Switch/2, Spring Kp/1
  Saturation/1 -> Normal/1
  Vz/1 -> Unary Minus1/1
  Spring Kp/1 -> Add/1
  Add/1 -> Switch/3
  Damper Kp/1 -> Add/2
  Switch/1 -> Saturation/1
  Z/1 -> Unary Minus/1
  Constant/1 -> Switch/1

== system UAV_Dynamics_Autopilot_Communication_ver2023b/Subsystem/Subsystem/Quadcopter Model1/Force and Moment Calculation/Rotor Model/Thrust model ==
  In1 : Inport
  Demux : Demux  Outputs=6
  Mux : Mux  Inputs=6
  Transfer Fcn{,1..5} (6 alike) : TransferFcn  Numerator=[rotorThrustMax]  Denominator=[rotorTimeConst 1]
  Out1 : Outport
  wires:
  Transfer Fcn5/1 -> Mux/6
  Transfer Fcn1/1 -> Mux/5
  Demux/6 -> Transfer Fcn5/1
  Demux/5 -> Transfer Fcn1/1
  In1/1 -> Demux/1
  Transfer Fcn/1 -> Mux/4
  Demux/2 -> Transfer Fcn3/1
  Demux/4 -> Transfer Fcn/1
  Transfer Fcn4/1 -> Mux/1
  Mux/1 -> Out1/1
  Demux/3 -> Transfer Fcn2/1
  Transfer Fcn2/1 -> Mux/3
  Demux/1 -> Transfer Fcn4/1
  Transfer Fcn3/1 -> Mux/2

== system UAV_Dynamics_Autopilot_Communication_ver2023b/Subsystem/Subsystem/Quadcopter Model1/Force and Moment Calculation/Rotor Model/Torque model ==
  In1 : Inport
  Demux : Demux  Outputs=6
  Mux : Mux  Inputs=6
  Transfer Fcn{1..6} (6 alike) : TransferFcn  Numerator=[rotorTorqueMax]  Denominator=[rotorTimeConst 1]
  Out1 : Outport
  wires:
  Transfer Fcn6/1 -> Mux/6
  Transfer Fcn5/1 -> Mux/5
  Demux/6 -> Transfer Fcn6/1
  Demux/5 -> Transfer Fcn5/1
  In1/1 -> Demux/1
  Transfer Fcn1/1 -> Mux/1
  Mux/1 -> Out1/1
  Demux/3 -> Transfer Fcn3/1
  Demux/4 -> Transfer Fcn4/1
  Demux/2 -> Transfer Fcn2/1
  Transfer Fcn2/1 -> Mux/2
  Transfer Fcn3/1 -> Mux/3
  Demux/1 -> Transfer Fcn1/1
  Transfer Fcn4/1 -> Mux/4

== system UAV_Dynamics_Autopilot_Communication_ver2023b/Subsystem/Subsystem/Quadcopter Model1/Force and Moment Calculation/Ground Model/Crash Detector/norm1 ==
  F : Inport
  Dot Product : DotProduct  OutDataTypeStr=Inherit: Inherit via internal rule
  Sqrt : Sqrt
  Out1 : Outport
  wires:
  Sqrt/1 -> Out1/1
  F/1 -> Dot Product/1, Dot Product/2
  Dot Product/1 -> Sqrt/1

== system UAV_Dynamics_Autopilot_Communication_ver2023b/Subsystem/Subsystem/Quadcopter Model1/Force and Moment Calculation/Ground Model/Friction Force/Soft Coulomb Friction ==
  note: Pennestrì, E., Rossi, V., Salvini, P. et al. Review and comparison of dry friction force models. Nonlinear Dyn 83, 1785–1801 (2016). https://doi.org/10.1007/s11071-015-2485-3
  In1 : Inport
  Tanh : Trigonometry  Operator=tanh
  friction coefficient : Gain  Gain=contact.translation.friction
  vd : Gain  Gain=1/contact.translation.vd
  Out1 : Outport
  wires:
  friction coefficient/1 -> Out1/1
  Tanh/1 -> friction coefficient/1
  vd/1 -> Tanh/1
  In1/1 -> vd/1

== system UAV_Dynamics_Autopilot_Communication_ver2023b/Subsystem/Subsystem/Quadcopter Model1/Force and Moment Calculation/Ground Model/Ground Moment Model/Soft Coulomb Friction ==
  note: Pennestrì, E., Rossi, V., Salvini, P. et al. Review and comparison of dry friction force models. Nonlinear Dyn 83, 1785–1801 (2016). https://doi.org/10.1007/s11071-015-2485-3
  In1 : Inport
  Tanh : Trigonometry  Operator=tanh
  friction coefficient : Gain  Gain=control.rotation.friction
  vd : Gain  Gain=1/control.rotation.vd
  Out1 : Outport
  wires:
  friction coefficient/1 -> Out1/1
  Tanh/1 -> friction coefficient/1
  vd/1 -> Tanh/1
  In1/1 -> vd/1

== matlab function UAV_Dynamics_Autopilot_Communication_ver2023b/Subsystem/Subsystem/Quadcopter Model1/Force and Moment Calculation/Rotor Model/MATLAB Function ==
  data: thrustEachRotor input; tauEachRotor input; rotorPositions input; netF output; netM output; rotorDir input
function [netF, netM] = getForceMoment(thrustEachRotor, tauEachRotor, rotorPositions, rotorDir)
%#codegen
Fx = 0;
Fy = 0;
Fz = -sum(thrustEachRotor);

netF = [Fx; Fy; Fz];

netM = [0; 0; 0]; %initialize
    for i = 1:6
        rotPos = rotorPositions(:, i);
        Fi = [0, 0, -thrustEachRotor(i)]';
        netM = netM +  cross(rotPos, Fi);%contribution from thrusts of each propeller
        netM(3) = netM(3) - rotorDir(i)*tauEachRotor(i); %contribution from counter torque acting on propeller
    end

end
